simulink model "slipWalking"  (R2014a)
settings: Solver=FixedStepDiscrete  StartTime=0.0  StopTime=inf  FixedStep=sample_time  RelTol=1e-3
libraries: slrtlib x5
settings Model: SimulationMode=external  BufferReuse=off  Creator=wmartin  LastModifiedBy=drl
settings SolverCC: EnableConcurrentExecution=on
settings DataIOCC: LimitDataPoints=off  MaxDataPoints=1e7  SaveFormat=StructureWithTime  SignalLogging=off  DSMLogging=off
settings OptimizationCC: BlockReduction=off  OptimizeBlockIOStorage=off  BufferReuse=off  GlobalBufferReuse=off  ExpressionFolding=off  ExpressionDepthLimit=2147483647  LocalBlockOutputs=off  SimCompilerOptimization=On
settings DebuggingCC: UnderspecifiedInitializationDetection=Classic  StateNameClashWarn=warning
settings HardwareCC: ProdIntDivRoundTo=Zero  ProdEndianess=LittleEndian  ProdHWDeviceType=Generic->32-bit x86 compatible
settings ModelReferenceCC: UpdateModelReferenceTargets=IfOutOfDate  ModelReferenceNumInstancesAllowed=Single  ModelReferenceMinAlgLoopOccurrences=on
settings RTWCC: SystemTargetFile=slrt.tlc  TemplateMakefile=slrt_default_tmf  Description=Simulink Real-Time  RTWVerbose=off  ProcessScript=slrt_make_rtw_hook  RTWCompilerOptimization=On
settings SimulinkRealTimeCC: GeneratePreprocessorConditionals=Disable all  EnableShiftOperators=on  RL32LogBufSizeModifier=1e8

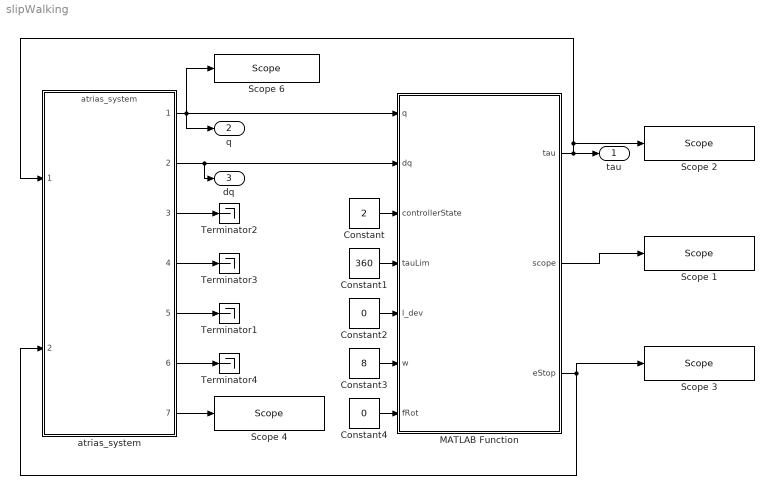
== system slipWalking ==
  Constant : Constant  Value=2
  Constant1 : Constant  Value=360
  Constant2 : Constant  Value=0
  Constant3 : Constant  Value=8
  Constant4 : Constant  Value=0
  MATLAB Function : MATLAB Function  TreatAsAtomicUnit=on
  Scope 1 : slrtlib/Displays and Logging/Scope   scopeno=4  scopetype=Target  autostart=on  viewmode=Numerical  formatstr='%15.6f'  grid=on  ylimits=[0,0]  nosamples=100  noprepostsamples=0  interleave=1  triggermode=FreeRun  triggersignal=1  trigsignalfromport=off  triggerlevel=0.0  triggerslope=Either  triggerscope=1  triggersample=0  filename=data.dat  mode=Lazy  writesize=512  autorestart=off  dynamicfilemode=off  maxwritefilesize=512*1024^2
  Scope 2 : slrtlib/Displays and Logging/Scope   scopeno=1  scopetype=Target  autostart=on  viewmode=Graphical sliding  formatstr='%15.6f'  grid=on  ylimits=[-600,600]  nosamples=100  noprepostsamples=0  interleave=1  triggermode=FreeRun  triggersignal=1  trigsignalfromport=off  triggerlevel=0.0  triggerslope=Either  triggerscope=1  triggersample=0  filename=data.dat  mode=Lazy  writesize=512  autorestart=off  dynamicfilemode=off  maxwritefilesize=512*1024^2
  Scope 3 : slrtlib/Displays and Logging/Scope   scopeno=2  scopetype=Target  autostart=on  viewmode=Numerical  formatstr='%d'  grid=on  ylimits=[0,0]  nosamples=100  noprepostsamples=0  interleave=1  triggermode=FreeRun  triggersignal=1  trigsignalfromport=off  triggerlevel=0.0  triggerslope=Either  triggerscope=1  triggersample=0  filename=data.dat  mode=Lazy  writesize=512  autorestart=off  dynamicfilemode=off  maxwritefilesize=512*1024^2
  Scope 4 : slrtlib/Displays and Logging/Scope   scopeno=5  scopetype=Target  autostart=on  viewmode=Numerical  formatstr='%d'  grid=on  ylimits=[0,0]  nosamples=100  noprepostsamples=0  interleave=1  triggermode=FreeRun  triggersignal=1  trigsignalfromport=off  triggerlevel=0.0  triggerslope=Either  triggerscope=1  triggersample=0  filename=data.dat  mode=Lazy  writesize=512  autorestart=off  dynamicfilemode=off  maxwritefilesize=512*1024^2
  Scope 6 : slrtlib/Displays and Logging/Scope   scopeno=3  scopetype=Target  autostart=on  viewmode=Numerical  formatstr='%15.6f'  grid=on  ylimits=[0,0]  nosamples=100  noprepostsamples=0  interleave=1  triggermode=FreeRun  triggersignal=1  trigsignalfromport=off  triggerlevel=0.0  triggerslope=Either  triggerscope=1  triggersample=0  filename=data.dat  mode=Lazy  writesize=512  autorestart=off  dynamicfilemode=off  maxwritefilesize=512*1024^2
  Terminator{1..4} (4 alike) : Terminator
  atrias_system : ModelReference  ModelNameDialog=atrias_system  SimulationMode=Normal  ModelReferenceVersion=1.1846  CopyOfModelName=atrias_system  DefaultDataLogging=on
  tau : Outport
  q : Outport  Port=2
  dq : Outport  Port=3
  wires:
  atrias_system/2 -> MATLAB Function/2(dq), dq/1
  MATLAB Function/1(tau) -> atrias_system/1, Scope 2/1, tau/1
  MATLAB Function/3(eStop) -> Scope 3/1, atrias_system/2
  atrias_system/3 -> Terminator2/1
  atrias_system/4 -> Terminator3/1
  atrias_system/5 -> Terminator1/1
  atrias_system/6 -> Terminator4/1
  Constant/1 -> MATLAB Function/3(controllerState)
  atrias_system/1 -> Scope 6/1, q/1, MATLAB Function/1(q)
  Constant1/1 -> MATLAB Function/4(tauLim)
  atrias_system/7 -> Scope 4/1
  MATLAB Function/2(scope) -> Scope 1/1
  Constant3/1 -> MATLAB Function/6(w)
  Constant2/1 -> MATLAB Function/5(l_dev)
  Constant4/1 -> MATLAB Function/7(fRot)

== matlab function slipWalking/MATLAB Function ==
  data: q input; tau output; scope output; dq input; controllerState input; eStop output; tauLim input; l_dev input; w input; fRot input
function [tau, scope, eStop] = slipWalkingController(q, dq, controllerState, tauLim, l_dev, w, fRot)
%SLIPWALKINGCONTROLLER Implements a self stable SLIP walking controller.
%
% Description:
%		A self stable walking controller based on ideas from the Spring Loaded
%		Inverted Pendulum reduced order model.
%
% Notes:
% 	- State indexes (rBl rBm rAl rAm lBl lBm lAl lAm rHm lHm bR bY bP)
%   - Input indexes (rB rA rH lB lA lH)
%
% Copyright 2014 Mikhail S. Jones

% Define default output argument values
eStop = false; % Emergency stop 
tau = zeros(6, 1); % Output torques

% Define constants
LEFT = 0; RIGHT = 1; % Stance leg
STAND = 0; WALK = 1; SHUTDOWN = 2; % Controller state
SINGLESUPPORT = 0; DOUBLESUPPORT = 1; % Walking state

% Define gait parameters
q1 = 3*pi/2 - deg2rad(67.678); % Stance leg angle at stance leg TD
q2 = 3*pi/2 - deg2rad(76.9143); % Stance leg angle at swing leg TO
q3 = 3*pi/2 - deg2rad(109.2973); % Stance leg angle at swing leg TD
q4 = 3*pi/2 - deg2rad(118.9815); % Stance leg angle at stance leg TO
s1 = 0;
s2 = (q2 - q1)/(q4 - q1);
s3 = (q3 - q1)/(q4 - q1);
s4 = 1;
l0 = 0.9; % Rest leg length
l_ret = 0.15; % Swing leg retraction

% Define actuator gains
kph = 1500; kdh = 25; % Hip actuators
kpl = 2000; kdl = 50; % Leg actuators
ks = 1600; % Spring constant

% Initialize persistent variables
persistent stanceLeg walkingState t_st t_sw q_exit l_exit;
if isempty(stanceLeg)
	% Define starting stance leg
	stanceLeg = LEFT;
	walkingState = SINGLESUPPORT;
	
	% Initialize timers
	t_st = 0;
	t_sw = 0;
    
    % Initial exit conditions
    q_exit = q4;
    l_exit = l0;
end % if

% Preallocate variables
q0 = zeros(4,1);
dq0 = zeros(4,1);

% Compute hip actuator torques using PD controller
tau([3 6]) = - q([9 10])*kph - dq([9 10])*kdh;

% Grab desired actuator states (torso, stance, swing)
switch stanceLeg
	case LEFT
		x = q([11 7 5 3 1 8 6 4 2]);
		dx = dq([11 7 5 3 1 8 6 4 2]);
    otherwise % RIGHT
		x = q([11 3 1 7 5 4 2 8 6]);
		dx = dq([11 3 1 7 5 4 2 8 6]);
end % switch

% Compute time invariant parameter
s = (x(1) + (x(2) + x(3))/2 - q1)/(q4 - q1);
ds = -(dx(1) + (dx(2) + dx(3))/2)/(q4 - q1);

% Bound time invariant parameter between 0 and 1 (or close to it)
s = clamp(s, 0, 1);
%ds = clamp(ds, 0, inf);

% Main controller state machine
switch controllerState
	case STAND
		% Desired position
		[q0(1), q0(2)] = legPos2MotorPos(q4, l0);
		[q0(3), q0(4)] = legPos2MotorPos(q2, l0);
		
		% Compute leg actuator torques using PD controller
		tau([2 1 5 4]) = (q0 - q([4 2 8 6]))*kpl - dq([4 2 8 6])*kdl;
		
	case WALK
		% Advance timers
		t_st = t_st + 0.001;
		t_sw = t_sw + 0.001;
		
		switch walkingState
			case SINGLESUPPORT
				% Compute desired stance leg state
				q_st = x(1) + (x(2) + x(3))/2;
				dq_st = dx(1) + (dx(2) + dx(3))/2;
				l_st = l0 + l_dev*sin(w*t_st);
				dl_st = l_dev*w*cos(w*t_st);
				
				% Compute desired swing leg state
                [q_sw, dq_sw] = cubic(s2, s3, q_exit, q1, 0, 0, s, ds); % -0.5, 1
                if s <= (s2 + s3)/2
                    [l_sw, dl_sw] = cubic(s2, (s2 + s3)/2, l_exit, l0 - l_ret, 0, 0, s, ds); % -1, 0
                else
                    [l_sw, dl_sw] = cubic((s2 + s3)/2, s3, l0 - l_ret, l0, 0, 0, s, ds); % 0, 0
                end % if

				% Check events
				if s >= s3
					walkingState = DOUBLESUPPORT;
					t_sw = t_st;
					t_st = 0;
				end % if

            otherwise % DOUBLESUPPORT
				% Compute desired stance leg state
				q_st = x(1) + (x(2) + x(3))/2;
				dq_st = dx(1) + (dx(2) + dx(3))/2;
				l_st = l0 + l_dev*sin(w*t_st);
				dl_st = l_dev*w*cos(w*t_st);

				% Compute desired swing leg state
				q_sw = x(1) + (x(4) + x(5))/2;
				dq_sw = dx(1) + (dx(4) + dx(5))/2;
				l_sw = l0 + l_dev*sin(w*t_sw);
				dl_sw = l_dev*w*cos(w*t_sw);

				% Check events
				if s >= s2
					walkingState = SINGLESUPPORT;
                    
					% Define cubic spline objects for swing leg angle
                    q_exit = q_sw;
                    l_exit = l_sw;
				end % if
		end % switch

		% Compute desired motor positions and velocities
		[q0(1), q0(2)] = legPos2MotorPos(q_st, l_st);
		[q0(3), q0(4)] = legPos2MotorPos(q_sw, l_sw);
		[dq0(1), dq0(2)] = legVel2MotorVel(l_st, dq_st, dl_st);
		[dq0(3), dq0(4)] = legVel2MotorVel(l_sw, dq_sw, dl_sw);

		% Compute actuator torques using PD controller
		switch stanceLeg
			case LEFT
				tau([5 4 2 1]) = (q0 - x(1) - q([8 6 4 2]))*kpl + (dq0 - dx(1) - dq([8 6 4 2]))*kdl;
                tau(5) = tau(5) + ks*(q(8) - q(7)) + fRot; % Feed forward term
                tau(4) = tau(4) + ks*(q(6) - q(5)) + fRot; % Feed forward term
			case RIGHT
				tau([2 1 5 4]) = (q0 - x(1) - q([4 2 8 6]))*kpl + (dq0 - dx(1) - dq([4 2 8 6]))*kdl;
                tau(2) = tau(2) + ks*(q(4) - q(3)) + fRot; % Feed forward term
                tau(1) = tau(1) + ks*(q(2) - q(1)) + fRot; % Feed forward term
		end % switch
		
		% Determine when to switch stance legs
		if s >= s3
			% Check which leg is the stance leg
			switch stanceLeg
				case LEFT; stanceLeg = RIGHT;
				case RIGHT; stanceLeg = LEFT;
			end % switch
		end % if
		
    otherwise % SHUTDOWN
		% Compute leg actuator torques using virtual damper
		tau = - dq([4 2 9 8 6 10]).*[kdl kdl kdh kdl kdl kdh].';
end % switch

% Limit currents
tau = clamp(tau, -tauLim, tauLim);

scope = [s; ds; walkingState; stanceLeg; q0];
end % slipWalkingController

function rad = deg2rad(deg)
%DEG2RAD Convert angles from degrees to radians

	rad = pi/180*deg;
end % deg2rad

function b = clamp(a, lim1, lim2)
%CLAMP Clamp value between two values.

	% Find which limit is min and max
	aMin = min(lim1);
	aMax = max(lim2);

	% Clamp value between limits
	b = max(min(a, aMax), aMin);
end % clamp

function [qA, qB] = legPos2MotorPos(q, l)
%LEGPOS2MOTORPOS Convert leg coordinates to motor coordinates

	qA = q - acos(l);
	qB = q + acos(l);
end % legPos2MotorPos

function [dqA, dqB] = legVel2MotorVel(l, dq, dl)
%LEGVEL2MOTORVEL Convert leg coordinates to motor coordinates

	dqA = dq + dl/sqrt(1 - l^2);
	dqB = dq - dl/sqrt(1 - l^2);
end % legVel2MotorVel

function [q, l] = motorPos2LegPos(qA, qB)
%MOTORPOS2LEGPOS Convert motor coordinates to leg coordinates

	q = (qA + qB)/2;
	l = cos((qA - qB)/2);
end % motorPos2LegPos

function [dq, dl] = motorVel2LegVel(qA, qB, dqA, dqB)
%MOTORVEL2LEGVEL Convert motor coordinates to leg coordinates

	dq = (dqA + dqB)/2;
    dl = -(sin((qA - qB)/2)*(dqA - dqB))/2;
end % motorVel2LegVel

function [y, dy] = cubic(x1, x2, y1, y2, dy1, dy2, x, dx)
%CUBIC Cubic spline interpolation.

    % Limit range since curve fit is only valid within range
    x = clamp(x, x1, x2);
    
    % Interpolate
    a0 = 2*(y1 - y2) + (dy1 + dy2)*(x2 - x1);
    a1 = y2 - y1 - dy1*(x2 - x1) - a0;
    a2 = dy1*(x2 - x1);
    a3 = y1;
    s = (x - x1)/(x2 - x1);
    y = a0*s^3 + a1*s^2 + a2*s + a3;
    dy = dx*(-3*a0*(x - x1)^2/(x1 - x2)^3 + 2*a1*(x - x1)/(x1 - x2)^2 - a2/(x1 - x2));
end % cubic
